simulink model "mavsim_trim"  (R2025b)
settings: Solver=ode45  StartTime=0.0  StopTime=30  MaxStep=0.05  RelTol=1e-6  AbsTol=1e-8
settings Model: Creator=ASUS  LastModifiedBy=ASUS

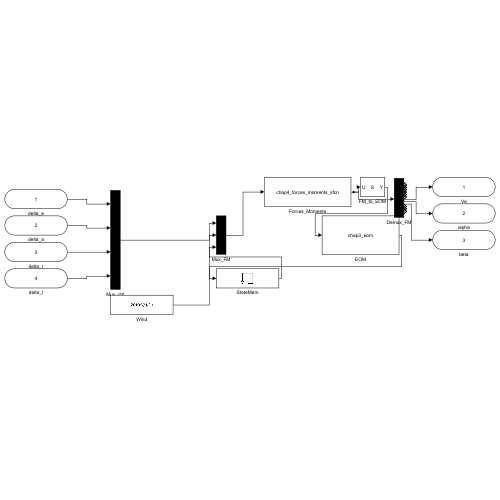
[thumbnail: Simulink's stored preview of the top-level diagram]
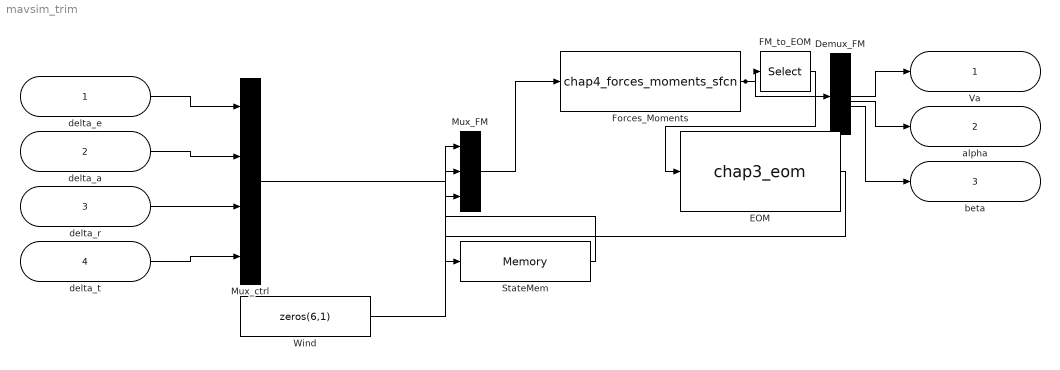
== system mavsim_trim ==
  delta_e : Inport
  delta_a : Inport  Port=2
  delta_r : Inport  Port=3
  delta_t : Inport  Port=4
  Demux_FM : Demux  Outputs=12
  EOM : M-S-Function  FunctionName=chap3_eom  Parameters=1212.16,25000,122200,139800,2200, 0,0,-1000, 352.486,-2.47782e-07,37.6435, -7.5423e-10,0.106391,0, 0,0,0
  FM_to_EOM : Selector  InputPortWidth=12  IndexOptions=Index vector (dialog)  Indices=1:6  OutputSizes=1
  Forces_Moments : M-S-Function  FunctionName=chap4_forces_moments_sfcn
  Mux_FM : Mux  Inputs=3
  Mux_ctrl : Mux
  StateMem : Memory  InitialCondition="[0,           0,       -1000,     352.486,-2.47782e-07,     37.6435, -7.5423e-10,    0.106391,           0,           0,           0,           0,]"
  Wind : Constant  Value=zeros(6,1)  OutDataTypeStr=double
  Va : Outport
  alpha : Outport  Port=2
  beta : Outport  Port=3
  wires:
  delta_e/1 -> Mux_ctrl/1
  delta_a/1 -> Mux_ctrl/2
  delta_r/1 -> Mux_ctrl/3
  delta_t/1 -> Mux_ctrl/4
  StateMem/1 -> Mux_FM/1
  Mux_ctrl/1 -> Mux_FM/2
  Wind/1 -> Mux_FM/3
  Mux_FM/1 -> Forces_Moments/1
  Forces_Moments/1 -> FM_to_EOM/1, Demux_FM/1
  FM_to_EOM/1 -> EOM/1
  EOM/1 -> StateMem/1
  Demux_FM/7 -> Va/1
  Demux_FM/8 -> alpha/1
  Demux_FM/9 -> beta/1
